simulink model "FIVELEVELFINAL"  (Simulink 7.3)
settings: Solver=ode3  StartTime=0.0  StopTime=0.5  FixedStep=1e-5  RelTol=1e-3
libraries: powerlib x43, simulink x4
settings Model: Creator=SAI GOWTHAM TEJA  LastModifiedBy=SAI GOWTHAM TEJA

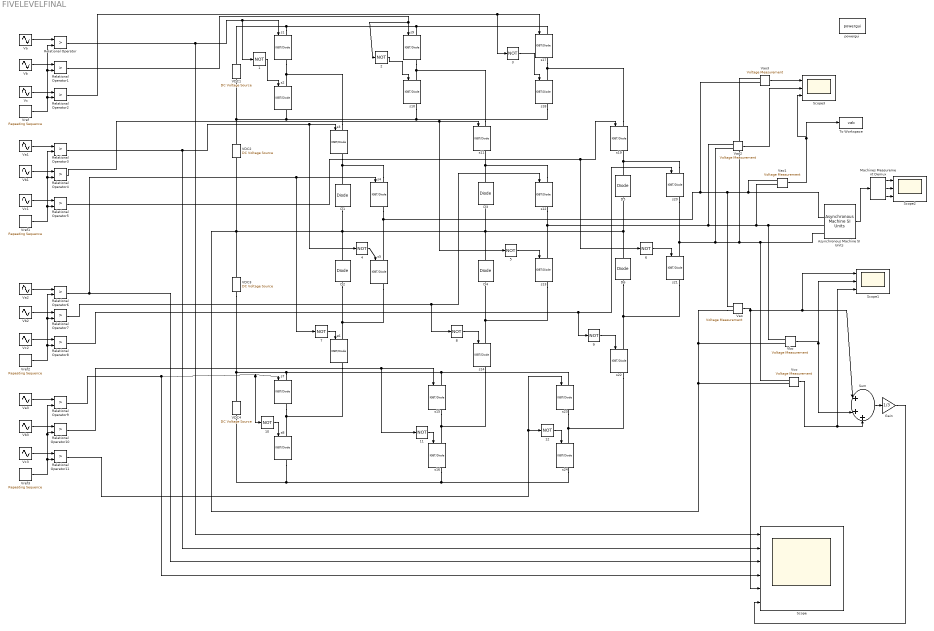
== system FIVELEVELFINAL ==
  {1..12} (12 alike) : Logic  Operator=NOT  AllPortsSameDT=off  OutDataTypeMode=boolean  LogicDataType=fixdt(0, 8)  OutDataTypeStr=boolean
  Asynchronous Machine SI Units : powerlib/Machines/Asynchronous Machine SI Units  DialogController=POWERSYS.PowerSysDialog  SystemSampleTime=-1  PresetModel="15:  5.4 HP (4KW)   400 V  50Hz 1430 RPM"  MechanicalLoad=Torque Tm  ShowDetailedParameters=on  RotorType=Squirrel-cage  ReferenceFrame=Stationary  NominalParameters=[4000 400 50]  Stator=[1.405 0.005839]  Rotor=[1.395 0.005839]  Lm=0.1722  Mechanical=[0.0131 0.002985 2]  PolePairs=2  InitialConditions=[1 0 0 0 0 0 0 0]  Units=SI  LoadFlowParameters=1492000  SimulateSaturation=off  Saturation=[14.03593122, 27.81365428, 53.79336849, 72.68890987, 97.98006896, 148.6815601, 215.7428561, 302.9841135, 428.7778367 ; 230, 322, 414, 460, 506, 552, 598, 644, 690]  TsPowergui=0  TsBlock=-1  IterativeModel=Forward Euler
  D{1..6} (6 alike) : powerlib/Power Electronics/Diode  DialogController=POWERSYS.PowerSysDialog  SystemSampleTime=-1  Ron=0.001  Lon=0  Vf=0.8  IC=0  UseSnubber=off  Rs=500  Cs=250e-9  Measurements=off
  Gain : Gain  Gain=1/3  ParameterDataType=fixdt(1, 16)  ParameterScaling=2^0  OutDataType=fixdt(1, 16)  OutScaling=2^0
  Machines Measurement Demux : powerlib/Machines/Machines Measurement Demux  DialogController=POWERSYS.PowerSysDialog  SystemSampleTime=-1  machType=Asynchronous  ssm1=on  ssm2=on  ssm3=on  ssm4=on  ssm5=on  ssm6=on  sm1=off  sm2=off  sm3=off  sm4=off  sm5=off  sm6=off  sm7=off  sm8=on  sm9=off  sm10=off  sm11=off  sm115=off  sm12=off  sm13=off  sm14=off  asm1=off  asm2=off  asm3=off  asm4=off  asm5=on  asm6=off  asm7=off  asm8=off  asm9=on  asm10=on  asm11=off  pmsm1=on  pmsm2=on  pmsm3=on  pmsm4=off  pmsm5=on  pmsm6=on  pmsm7=on  lastType=1
  Relational Operator{,1..11} (12 alike) : RelationalOperator  Operator=>  LogicOutDataTypeMode=boolean  LogicDataType=fixdt(0, 8)  OutDataTypeStr=boolean
  Scope : Scope  NumInputPorts=6
      settings: YMin=-5~-5~-5~-5~-150~-5  YMax=5~5~5~5~150~5
  Scope1 : Scope  NumInputPorts=3
      settings: YMin=-5~-5~-5  YMax=5~5~5
  Scope2 : Scope  NumInputPorts=3
      settings: YMin=-5~-5~-5  YMax=5~5~5  SaveName=ScopeData2
  Scope3 : Scope  NumInputPorts=3
      settings: YMin=-5~-5~-5  YMax=5~5~5  SaveName=ScopeData3
  Sum : Sum  Inputs=|+++  OutDataType=fixdt(1, 16)  OutScaling=2^0
  To Workspace : ToWorkspace  VariableName=vab  SampleTime=-1  SaveFormat=Structure With Time
  VDC{1..4} (4 alike) : powerlib/Electrical Sources/DC Voltage Source  DialogController=POWERSYS.PowerSysDialog  SystemSampleTime=-1  Amplitude=127.5  Measurements=None
  Va : Sin  Amplitude=0.9  Bias=0  Frequency=2*pi*50  Phase=0  Samples=10  SampleTime=0  Offset=0
  Va1 : Sin  Amplitude=0.9  Bias=0  Frequency=2*pi*50  Phase=0  Samples=10  SampleTime=0  Offset=0
  Va2 : Sin  TimeSource=Use external signal  Amplitude=0.9  Bias=0  Frequency=2*pi*50  Phase=0  Samples=10  SampleTime=0  Offset=0
  Va3 : Sin  Amplitude=0.9  Bias=0  Frequency=2*pi*50  Phase=0  Samples=10  SampleTime=0  Offset=0
  Vao{,1..3} (4 alike) : powerlib/Measurements/Voltage Measurement  DialogController=POWERSYS.PowerSysDialog  SystemSampleTime=-1  PhasorSimulation=off  OutputType=Complex  PSBequivalent=0
  Vb{,1..3} (4 alike) : Sin  Amplitude=0.9  Bias=0  Frequency=2*pi*50  Phase=-2*pi/3  Samples=10  SampleTime=0  Offset=0
  Vbo : powerlib/Measurements/Voltage Measurement  DialogController=POWERSYS.PowerSysDialog  SystemSampleTime=-1  PhasorSimulation=off  OutputType=Complex  PSBequivalent=0
  Vc{,1..3} (4 alike) : Sin  Amplitude=0.9  Bias=0  Frequency=2*pi*50  Phase=-4*pi/3  Samples=10  SampleTime=0  Offset=0
  Vco : powerlib/Measurements/Voltage Measurement  DialogController=POWERSYS.PowerSysDialog  SystemSampleTime=-1  PhasorSimulation=off  OutputType=Complex  PSBequivalent=0
  Vref : simulink/Sources/Repeating Sequence  SystemSampleTime=-1  rep_seq_t=[0 0.5/3000 1/3000]  rep_seq_y=[0.5 1 0.5]
  Vref1 : simulink/Sources/Repeating Sequence  SystemSampleTime=-1  rep_seq_t=[0 0.5/3000 1/3000]  rep_seq_y=[0 0.5 0]
  Vref2 : simulink/Sources/Repeating Sequence  SystemSampleTime=-1  rep_seq_t=[0 0.5/3000 1/3000]  rep_seq_y=[-0.5 0 -0.5]
  Vref3 : simulink/Sources/Repeating Sequence  SystemSampleTime=-1  rep_seq_t=[0 0.5/3000 1/3000]  rep_seq_y=[-1 -0.5 -1]
  powergui : powerlib/powergui  Priority=1  SystemSampleTime=-1  SimulationMode=Continuous  SampleTime=50e-6  frequency=60  SPID=off  DisableSnubberDevices=off  DisableRonSwitches=off  DisableVfSwitches=off  SwTol=0  Interpol=off  frequencyindice=0  echomessages=off  HookPort=off  DisplayEquations=off  FunctionMessages=off  EnableUseOfTLC=off  x0status=blocks  RestoreLinks=warning  Frange=[0:2:500]  Ylog=off  Xlog=on  ShowGrid=off  save=off  variable=ZData  structure=vab  ZoomFFT=off  StartTime=0.3  cycles=1  DisplayStyle=1  fundamental=50  FreqAxis=off  MaxFrequency=9000  frequencyindicesteady=1  RmsSteady=1  display=off  Ts=0  methode=off
  s{1..24} (24 alike) : powerlib/Power Electronics/IGBT//Diode  DialogController=POWERSYS.PowerSysDialog  SystemSampleTime=-1  Ron=1e-3  Rs=1e5  Cs=inf  Measurements=on
  wires:
  Va/1 -> Relational Operator/1
  Vb/1 -> Relational Operator1/1
  Vc/1 -> Relational Operator2/1
  Vref/1 -> Relational Operator/2, Relational Operator1/2, Relational Operator2/2
  Va1/1 -> Relational Operator3/1
  Vb1/1 -> Relational Operator4/1
  Vc1/1 -> Relational Operator5/1
  Vref1/1 -> Relational Operator3/2, Relational Operator4/2, Relational Operator5/2
  Va2/1 -> Relational Operator6/1
  Vb2/1 -> Relational Operator7/1
  Vc2/1 -> Relational Operator8/1
  Vref2/1 -> Relational Operator6/2, Relational Operator7/2, Relational Operator8/2
  Va3/1 -> Relational Operator9/1
  Vb3/1 -> Relational Operator10/1
  Vc3/1 -> Relational Operator11/1
  Vref3/1 -> Relational Operator9/2, Relational Operator10/2, Relational Operator11/2
  Relational Operator/1 -> s1/1, 1/1, Scope/1
  Relational Operator1/1 -> s9/1, 2/1
  Relational Operator2/1 -> s17/1, 3/1
  1/1 -> s2/1
  2/1 -> s10/1
  3/1 -> s18/1
  Relational Operator3/1 -> s3/1, 4/1, Scope/2
  Relational Operator4/1 -> s11/1, 5/1
  Relational Operator5/1 -> s19/1, 6/1
  4/1 -> s5/1
  5/1 -> s13/1
  6/1 -> s21/1
  Relational Operator6/1 -> Scope/3, s4/1, 7/1
  Relational Operator7/1 -> s12/1, 8/1
  Relational Operator8/1 -> s20/1, 9/1
  7/1 -> s6/1
  8/1 -> s14/1
  9/1 -> s22/1
  Relational Operator9/1 -> s7/1, 10/1, Scope/4
  Relational Operator10/1 -> s15/1, 11/1
  Relational Operator11/1 -> s23/1, 12/1
  10/1 -> s8/1
  11/1 -> s16/1
  12/1 -> s24/1
  Vao/1 -> Scope/5, Sum/1, Scope1/1
  Machines Measurement Demux/1 -> Scope2/1
  Machines Measurement Demux/2 -> Scope2/2
  Machines Measurement Demux/3 -> Scope2/3
  Asynchronous Machine SI Units/1 -> Machines Measurement Demux/1
  Vbo/1 -> Sum/2, Scope1/2
  Vco/1 -> Sum/3, Scope1/3
  Sum/1 -> Gain/1
  Vao1/1 -> To Workspace/1, Scope3/3
  Vao3/1 -> Scope3/1
  Vao2/1 -> Scope3/2
  Gain/1 -> Scope/6
  connections:
  s1/LConn1 -- s9/LConn1 -- s17/LConn1 -- VDC1/RConn1
  s3/LConn1 -- s1/RConn1 -- s2/LConn1
  s4/LConn1 -- s3/RConn1 -- D1/RConn1
  s4/RConn1 -- s5/LConn1 -- Asynchronous Machine SI Units/LConn1 -- Vao1/LConn1 -- Vao/LConn1 -- Vao3/LConn2
  Vao/LConn2 -- D4/RConn1 -- D5/LConn1 -- D6/RConn1 -- D3/LConn1 -- D1/LConn1 -- D2/RConn1 -- VDC2/LConn1 -- VDC3/RConn1 -- Vco/LConn2 -- Vbo/LConn2
  s5/RConn1 -- D2/LConn1 -- s6/LConn1
  s18/RConn1 -- s10/RConn1 -- VDC1/LConn1 -- VDC2/RConn1 -- s2/RConn1
  s7/LConn1 -- s15/LConn1 -- s23/LConn1 -- VDC3/LConn1 -- VDC4/RConn1
  s24/RConn1 -- s16/RConn1 -- s8/RConn1 -- VDC4/LConn1
  s6/RConn1 -- s7/RConn1 -- s8/LConn1
  s11/LConn1 -- s9/RConn1 -- s10/LConn1
  s12/LConn1 -- D3/RConn1 -- s11/RConn1
  s12/RConn1 -- s13/LConn1 -- Asynchronous Machine SI Units/LConn2 -- Vbo/LConn1 -- Vao1/LConn2 -- Vao2/LConn1
  s13/RConn1 -- s14/LConn1 -- D4/LConn1
  s14/RConn1 -- s15/RConn1 -- s16/LConn1
  s19/LConn1 -- s17/RConn1 -- s18/LConn1
  s20/LConn1 -- D5/RConn1 -- s19/RConn1
  s20/RConn1 -- s21/LConn1 -- Vao2/LConn2 -- Asynchronous Machine SI Units/LConn3 -- Vco/LConn1 -- Vao3/LConn1
  s21/RConn1 -- D6/LConn1 -- s22/LConn1
  s22/RConn1 -- s23/RConn1 -- s24/LConn1
